simulink model "Ejer15_PesoIdeal"  (R2023b)
settings: Solver=FixedStepDiscrete  StartTime=0  StopTime=52  FixedStep=1  RelTol=1e-3
undefined symbols (not defined in the file): ejercicio, metabolismo, P0
settings Model: Creator=alfre  LastModifiedBy=alfre

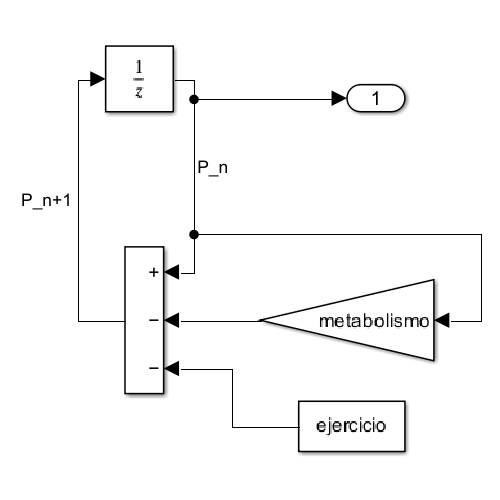
[thumbnail: Simulink's stored preview of the top-level diagram]
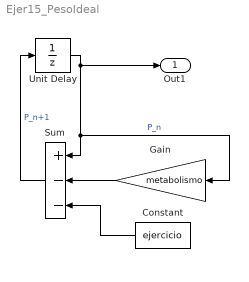
== system Ejer15_PesoIdeal ==
  Constant : Constant  Value=ejercicio
  Gain : Gain  Gain=metabolismo
  Sum : Sum  Inputs=+--
  Unit Delay : UnitDelay  InitialCondition=P0  SampleTime=-1  HasFrameUpgradeWarning=on
  Out1 : Outport
  wires:
  Sum/1 -> Unit Delay/1  "P_n+1"
  Unit Delay/1 -> Out1/1, Sum/1, Gain/1  "P_n"
  Gain/1 -> Sum/2
  Constant/1 -> Sum/3
